simulink model "VisualLocalizationAgent"  (R2024b)
settings: Solver=FixedStepAuto  StartTime=0.0  StopTime=inf  FixedStep=0.005  RelTol=1e-3  EnableMultiTasking=on
undefined symbols (not defined in the file or in its folder): DiscIntNeverNeededParam, gray, Sim3dSensor
libraries: robotcorelib x7, dspstat3 x3, eeGeneralControl x2, sim3dcameralib x1, sim3dlib x1, uavsim3dlib x1, uavutilslib x1
settings Model: Creator=The MathWorks, Inc.  LastModifiedBy=Sasha
settings SolverCC: AlgebraicLoopSolver=TrustRegion  PositivePriorityOrder=on  AutoInsertRateTranBlk=on  MaxZcPerStep=1
settings OptimizationCC: DefaultParameterBehavior=Inlined  EnhancedBackFolding=on  PassReuseOutputArgsAs=Individual arguments  ZeroExternalMemoryAtStartup=off  ZeroInternalMemoryAtStartup=off  MaxStackSize=200000  OptimizeBlockOrder=speed  DifferentSizesBufferReuse=on  OptimizationCustomize=off  EfficientTunableParamExpr=on
settings DebuggingCC: ParameterTunabilityLossMsg=error  UnconnectedInputMsg=warning  UnconnectedOutputMsg=warning  UnconnectedLineMsg=warning  SymbolicDimsDataTypeCodeGenerationDiagnostic=none
settings HardwareCC: ProdBitPerPointer=32  ProdBitPerSizeT=32  ProdBitPerPtrDiffT=32  ProdLargestAtomicInteger=Long  ProdLargestAtomicFloat=Double  ProdWordSize=32  ProdLongLongMode=on  ProdHWDeviceType=ARM Compatible->ARM Cortex-A (32-bit)
settings ModelReferenceCC: EnableRefExpFcnMdlSchedulingChecks=on
settings RTWCC: Description=Embedded Coder  SystemTargetFile=ert.tlc  HardwareBoard=Raspberry Pi  TLCOptions="-aInlineSetEventsForThisBaseRateFcn=TLC_FALSE -aSuppressMultiTaskScheduler=TLC_FALSE  -aRateBasedStepFcn=0"  TemplateMakefile=ert_default_tmf  Toolchain=GNU GCC Embedded Linux  BuildConfiguration=Faster Runs  GPUComputeCapability=3.5  DLArmComputeVersion=19.05
settings CodeAppCC: ForceParamTrailComments=on  IgnoreCustomStorageClasses=off  OperatorAnnotations=on  SimulinkDataObjDesc=on  SFDataObjDesc=on  InsertBlockDesc=on
settings ERTTargetCC: CodeReplacementLibrary=ARM Cortex-A CMSIS  SupportVariableSizeSignals=on  ExtModeTransport=2  ExtModeStaticAlloc=on  ExtModeMexFile=ext_xcp  ExtModeIntrfLevel=Level2 - Open

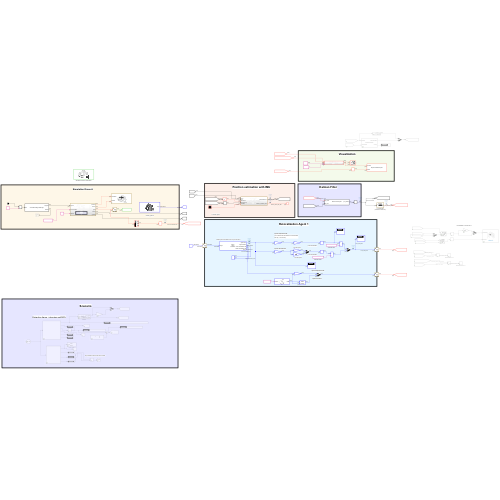
[thumbnail: Simulink's stored preview of the top-level diagram]
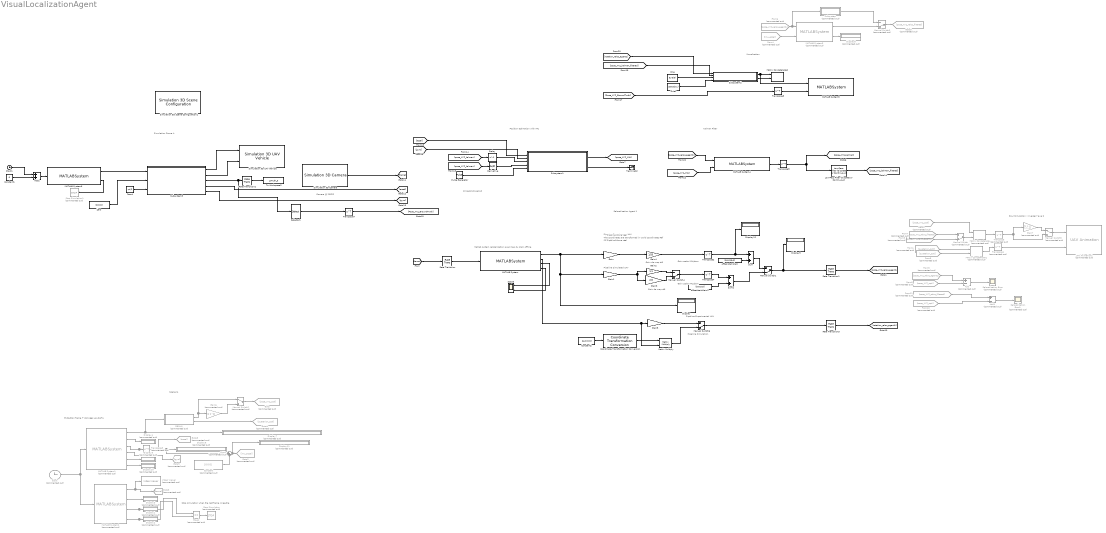
== system VisualLocalizationAgent ==
  note: Stop simulation when the last frame is reache
  note: Gain de map #6
  note: Pour Simulation : Inverser l'axe Z
  note: Pipeline Experimental UAV
  note: Matlab system relocalisation avec map du slam offline
  note: Gain scale IMU/slam
  note: Extraction frame + données uavDATA
  note: The coordinates are transformed in world coordinates
      |
      | Ref opti : (Y et Z inversé)
  note: Gain scale IMU/slam
  note: Pipeline drone réel
  note: Pipeline drone réel
  note: Pipeline Simulated UAV
  note: Gain de map #8
  note: 10 seconds period
  note: Relocalization Agent 1
  note: Scenario
  note: Position estimation with IMU
  note: Kalman Filter
  note: Visualization
  note: Camera @ 20FPS
  note: Simulation Drone A
  note: Pipeline Experimental UAV
  note: Pipeline Simulation
  Add : Sum  Commented=on  Inputs=+-
  Add1 : Sum  Commented=on  Inputs=+-
  Add2 : Sum
  Clock : Clock  Commented=on
  Clock1 : Clock
  Constant : Constant  Commented=on  Value=[0 0 0]
  Constant1 : Constant  Value=0
  Constant2 : Constant  Value=[pi/2;0;0]
  Coordinate Transformation Conversion : robotcorelib/Coordinate Transformation Conversion  InputRepresentation=Euler Angles  InputEulerSequence=ZYX  ShowTrVecInputPort=on  OutputRepresentation=Rotation Matrix  OutputEulerSequence=ZYX  ShowTrVecOutputPort=on  SimulateUsing=Code generation
  DEMUX : Subsystem  Commented=on
  Delay : Delay  DelayLength=1  InitialCondition=[0;0;0]
  Derivative : Derivative
  Display : Display
  Display{1..8,10..11} (10 alike) : Display  Commented=on
  Display12 : Display
  Display9 : Display
  Equal : RelationalOperator  Commented=on  Operator===  OutDataTypeStr=boolean  RndMeth=Simplest  InputSameDT=off
  From1 : From  Commented=on  GotoTag=quaterion_opti
  From10 : From  Commented=on  GotoTag=pose_XYZ_opti
  From11 : From  Commented=on  GotoTag=pose_XYZ_reloc_filtered
  From2 : From  Commented=on  GotoTag=pose_XYZ_opti
  From3 : From  Commented=on  GotoTag=pose_XYZ_reloc_agent1
  From4 : From  Commented=on  GotoTag=imu_accel
  From5 : From  Commented=on  GotoTag=quaterion_opti
  From6 : From  Commented=on  GotoTag=pose_XYZ_reloc_agent1
  From7 : From  Commented=on  GotoTag=pose_XYZ_reloc_filtered
  From8 : From  Commented=on  GotoTag=pose_XYZ_opti
  From9 : From  Commented=on  GotoTag=pose_XYZ_reloc_agent1
  Gain : Gain  Gain=[1 0 0; 0 -1 0 ; 0 0 -1]  Multiplication=Matrix(u*K)
  Gain1 : Gain  Gain=[0 -1 0; 1 0 0 ; 0 0 1]  Multiplication=Matrix(u*K)
  Gain2 : Gain  Gain=1.1
  Gain3 : Gain  Gain=2.6
  Gain4 : Gain  Gain=1/20
  Gain5 : Gain  Gain=[1 0 0; 0 -1 0 ; 0 0 -1]  Multiplication=Matrix(u*K)
  Gain6 : Gain  Commented=on  Gain=[1 1 -1]
  Gain7 : Gain  Commented=on  Gain=[1 1 -1; 1 1 -1]
  Goto : Goto  Commented=on  GotoTag=pose_XYZ_opti
  Goto2 : Goto  Commented=on  GotoTag=imu_accel
  Goto3 : Goto  Commented=on  GotoTag=frame
  Goto4 : Goto  Commented=on  GotoTag=quaterion_opti
  Goto5 : Goto  Commented=on  GotoTag=pose_XYZ_reloc_filtered
  Goto8 : Goto  Commented=on  GotoTag=accel
  Goto9 : Goto  Commented=on  GotoTag=gyro
  Low-Pass Filter (Discrete or Continuous) : eeGeneralControl/Low-Pass Filter (Discrete or Continuous)  K=1  T=0.05  B=inf  A=-inf  init_option=Inherited from block input  x0=0  Ts=-1
  MATLAB System : MATLABSystem  System=Modif_of_HelperVisualLocalizationSystem  FocalLength=[1109,1109]  PrincipalPoint=[640,360]  ImageSize=[720,1280]  ScaleFactor=1.2  NumLevels=8  NumPoints=2000  XLim=[-100 100]  YLim=[-100 100]  ZLim=[-100 100]  SampleTime=0.1  ScenariosDirectory=C:\Users\vince\Documents\SEN5\CollaborativeSLAM\Scenarios  ScenarioName=8
      mask Type: Modif_of_HelperVisualLocalizationSystem
      mask Display:
      | disp(['Helper' char(10) 'Visual' char(10) 'Localization']);
      | port_label('input',1,'Image');
      | port_label('output',1,'Agent Pose');
      | port_label('output',2,'Agent Rotation');
      | port_label('output',3,'Local relocalization fail');
      | port_label('output',4,'Global relocalization fail');
  MATLAB System1 : MATLABSystem  Commented=on  System=GTruthPlayerSystem  groundTruthFile=C:\Users\vince\Documents\SEN5\CollaborativeSLAM\Scenarios\7\uavData.mat  SimulateUsing=Interpreted execution
  MATLAB System2 : MATLABSystem  Commented=on  System=ImagePlayerSystem  imageFolder=C:\Users\vince\Documents\SEN5\CollaborativeSLAM\Scenarios\7\images  cameraSize=[720,1280, 1]  groundTruthFile=C:\Users\vince\Documents\SEN5\CollaborativeSLAM\Scenarios\7\uavData.mat  SimulateUsing=Interpreted execution
  MATLAB System3 : MATLABSystem  Commented=on  System=PositionAccelFilter  maxPositionJump=0.2  maxAcceleration=10.0  windowSize=5  alpha=0.1  SimulateUsing=Code generation
      mask Type: PositionAccelFilter
      mask Display:
      | disp('PositionAccelFilter');
      | port_label('input',1,'position');
      | port_label('input',2,'acceleration');
      | port_label('output',1,'filteredPosition');
      | port_label('output',2,'isJump');
  MATLAB System4 : MATLABSystem  System=KalmanFusionSystem  dt=0.1  noise_std=0.1  Q=0.001 * eye( 6 )  R=diag( [ 0.3, 0.3, 0.3, 0.1, 0.1, 0.1 ] )  SimulateUsing=Interpreted execution
  MATLAB System5 : MATLABSystem  System=HelperVisualizationSystem  XLim=[-10 50]  YLim=[-10 10]  ZLim=[-10 10]  SampleTime=-1  ScenariosDirectory=C:\Users\vince\Documents\SEN5\CollaborativeSLAM\Scenarios  ScenarioName=8  NumberOfPoses=1  SimulateUsing=Interpreted execution
      mask Type: HelperVisualizationSystem
      mask Display:
      | disp('HelperVisualizationSystem');
      | port_label('input',1,'TformID');
      | port_label('input',2,'Gtruth');
  MATLAB System6 : MATLABSystem  System=SmoothBasicWaypointManager  ScenariosDirectory=C:\Users\vince\Documents\SEN5\CollaborativeSLAM\Scenarios  ScenarioName=9a  StepTime=0.01  SimulateUsing=Interpreted execution
  Manual Switch : ManualSwitch  Commented=on  CurrentSetting=0
  Manual Switch1 : ManualSwitch  CurrentSetting=0
  Manual Switch2 : ManualSwitch  Commented=on
  Manual Switch3 : ManualSwitch  Commented=on  CurrentSetting=0
  Manual Switch4 : ManualSwitch  CurrentSetting=0
  Manual Switch5 : ManualSwitch  Commented=on
  Manual Switch6 : ManualSwitch  CurrentSetting=0
  Matrix Concatenate : Concatenate  Commented=on  Mode=Multidimensional array  ConcatenateDimension=2
  Matrix Concatenate1 : Concatenate  Commented=on  Mode=Multidimensional array  ConcatenateDimension=2
  Matrix Concatenate2 : Concatenate  Mode=Multidimensional array  ConcatenateDimension=2
  Matrix Multiply : Product  Multiplication=Matrix(*)
  One : Constant  Value=eye(3)  OutDataTypeStr=Inherit: Inherit via back propagation
  One1 : Constant  Value=zeros(3,1)  OutDataTypeStr=Inherit: Inherit via back propagation
  Pulse Generator : DiscretePulseGenerator  PulseType=Time based  Period=0.05  PulseWidth=50
  Rate Transition : RateTransition
  Rate Transition1 : RateTransition
  Rate Transition2 : RateTransition  OutPortSampleTime=0.01
  Rate Transition3 : RateTransition
  Relocalization Error : Scope  Commented=on
  Relocalization Error1 : Scope  Commented=on
  Scope : Scope  NumInputPorts=2
  Selector1 : Selector  InputPortWidth=7  IndexOptions=Index vector (dialog)  Indices=[1 2 3]  OutputSizes=1
  Simulation 3D Camera : sim3dcameralib/Simulation 3D Camera  Priority=1  sensorTag=Sim3dSensor�  sensorId=1  sensorName=Sim3dSensor�  vehTagList={'Scene Origin';'SimulinkVehicle1'}  vehTag=SimulinkVehicle1  mountLoc=Origin  offsetFlag=on  tmountOffset=[0.1, 0, 0.1]  extTmount=off  rmountOffset=[0, 0, 0]  extRmount=off  FocalLength=[1109, 1109]  OpticalCenter=[640, 360]  ImageSize=[720, 1280]  RadialDistortion=[0, 0]  TangentialDistortion=[0, 0]  SensorSkew=0  DepthOutportEnabled=off  SemanticOutportEnabled=off  TransformOutportEnabled=off  SampleTime=1/20  mountPoint=[0.1 0 0.1]  mountOrientation=[0 0 0]  aMode=3  ID=1
      settings: LibrarySourceBlock=drivingsim3d/Simulation 3D Camera
  Simulation 3D Scene Configuration1 : sim3dlib/Simulation 3D Scene Configuration  Priority=0  ProjectFormat=Default Scenes  SceneDesc=US city block  ProjectName=D:\Program Files\MATLAB\R2024b\toolbox\shared\sim3d_projects\automotive_project_windows\UE\WindowsNoEditor\VehicleSimulation.exe  ScenePath=/Game/Maps/USCityBlock  EnableOpenDRIVE=off  vehTagList={'Scene Origin';'SimulinkVehicle1'}  vehTag=SimulinkVehicle1  FreeCameraInitialTranslation=[0, 0, 0]  FreeCameraDefaultInitialTranslation=[-6, 0, 2]  FreeCameraInitialRotation=[0, 0, 0]  FreeCameraDefaultInitialRotation=[0, -15, 0]  OpVisEn=off  Ts=1/100  EnableWindow=on  EnableRemoteAccess=off  EnableWeather=off  SunAzimuth=90  SunAltitude=40.0  EnableGeospatialSun=off  Latitude=0  Longitude=0  Date=2023-01-01  Time=10:30:00  GeoTimeZone=-5.0  SunDaylightSaving=off  wind=1  clouds=10  EnableVolumetricClouds=off  CloudCoverage=0  CloudAltitude=6  fog=0  rain=0  RaindropsEffect=off  SnowDensity=0  EnableGeospatial=off  UseTrueOrigin=off  OriginHeight=200  OriginLatitude=40.744652  OriginLongitude=-73.988864  MapStyle=Aerial  AdditionalAssetIDs=[]  UseAdvancedSunSky=off  SolarTime=11  TimeZone=-5  Day=21  Month=9  Year=2022  UseDaylightSavingTime=on  DSTStartDay=10  DSTStartMonth=3  DSTEndDay=3  DSTEndMonth=11  DSTSwitchHour=2  sensorTag=MainCamera1  sensorId=1  sensorName=MainCamera1  mountLoc=Origin  offsetFlag=off  tmountOffset=[0, 0, 0]  rmountOffset=[0, 0, 0]  HorizontalResolution=1280  VerticalResolution=720  HorizontalFOV=60  mountPoint=[0 0 0]  mountOrientation=[0 0 0]  aMode=4  ID=1  GeoTrigger=Inactive
      settings: LibrarySourceBlock=uavsim3dlib/Simulation 3D Scene Configuration
  Simulation 3D UAV Vehicle : uavsim3dlib/Simulation 3D UAV Vehicle  Priority=-1  Mesh=Quadrotor  MeshPath=/MathWorksUAVContent/UAVs/HexaRotorUAV/HexaRotor.HexaRotor  Color=Black  ActorName=SimulinkVehicle1  UseGlobalFrame=off  InitialTranslation=[0 0 0]  InitialRotation=[0 0 0]  InitialTranslationGlobal=[0 0 0]  InitialGeoOrigin=[0 0 0]  InitialRotationGlobal=[0 0 0]  SampleTime=1/100  ActorType=SimulinkVehicle  ID=1  aMode=4  ActorTag=SimulinkVehicle1
  Stop Simulation : Stop  Commented=on
  Stop Simulation1 : Stop  Commented=on
  Subsystem : Subsystem  Commented=on
  Subsystem1 : Subsystem
  Subsystem2 : Subsystem
  Subsystem3 : Subsystem
  Sum : Sum
  Sum1 : Sum  Commented=on  Inputs=|++
  Sum2 : Sum
  Terminator : Terminator
  To Workspace2 : ToWorkspace  VariableName=gTruth_a  SaveFormat=Timeseries  SampleTime=-1
  Transpose : Math  Commented=on  Operator=transpose
  Transpose1 : Math  Commented=on  Operator=transpose
  Transpose{2,4..5,7..8} (5 alike) : Math  Operator=transpose
  Transpose3 : Math  Commented=on  Operator=transpose
  UAV Animation1 : uavutilslib/UAV Animation  Commented=on  NumUAV=2  DynamicUAVConfig=off  UAVType=Multirotor  UAVSize=0.1  UAVColor=[1 0 0]  UAVTrajectoryAlpha=1  InertialZDirection=Down  RotationFormat=Quaternion  DrawMarkers=off  SampleTime=-1
  Video Viewer : VideoViewer  Commented=on  colormapValue=gray(256)  FigPos=[184.333333333333 766.666666666667 706 510]
  Zero : Constant  Value=[0;0;0]  OutDataTypeStr=Inherit: Inherit via back propagation
  Zero4 : Constant  Value=-pi/2  OutDataTypeStr=Inherit: Inherit via back propagation
  offset start slam : Constant  Value=[0;0.33;0]
  offset start slam1 : Constant  Value=[0;0;3.5]
  wires:
  MATLAB System2/1 -> Goto3/1, Video Viewer/1
  MATLAB System/2 -> Matrix Multiply/2, Gain5/1  "Agent_Rotation"
  MATLAB System/1 -> Gain1/1, Display/1, Gain/1  "Agent_Translation_reloc"
  MATLAB System/3 -> Scope/1  "Local relocalization fail"
  MATLAB System/4 -> Scope/2  "Global relocalization fail"
  MATLAB System2/3 -> Equal/1, Display1/1
  Clock/1 -> MATLAB System2/1, MATLAB System1/1
  MATLAB System2/4 -> Equal/2, Display2/1
  MATLAB System2/2 -> Display3/1
  MATLAB System1/1 -> Display7/1, DEMUX/1(pose_refopti_gtruth)
  offset start slam/1 -> Sum/2
  Matrix Concatenate/1 -> Transpose/1
  Matrix Concatenate1/1 -> Transpose1/1
  Transpose/1 -> Gain7/1, Manual Switch5/2
  Transpose1/1 -> UAV Animation1/2
  From3/1 -> Manual Switch/2
  DEMUX/1(XYZ_gtruth) -> Manual Switch2/1, Gain6/1
  MATLAB System1/2 -> Display4/1
  MATLAB System1/5 -> Display5/1
  MATLAB System1/6 -> Display10/1
  MATLAB System1/3 -> Goto8/1, Transpose3/1
  Gain/1 -> Gain4/1
  Gain4/1 -> Transpose2/1
  Transpose2/1 -> Display12/1, Sum/1
  DEMUX/2(quaterion_gtruth) -> Goto4/1
  From1/1 -> Matrix Concatenate1/1
  From5/1 -> Matrix Concatenate1/2
  From4/1 -> MATLAB System3/2
  From6/1 -> Subsystem/1(In1), MATLAB System3/1
  From7/1 -> Manual Switch/1
  Manual Switch/1 -> Matrix Concatenate/2
  Transpose3/1 -> Sum1/1, Display6/1
  MATLAB System3/2 -> Display8/1
  Constant/1 -> Sum1/2
  Sum1/1 -> Display11/1, Goto2/1
  Sum/1 -> Manual Switch1/1
  MATLAB System3/1 -> Manual Switch3/2
  Subsystem/1(Out1) -> Manual Switch3/1
  Manual Switch1/1 -> Display9/1, Rate Transition1/1  "Pose_XYZ_Reloc"
  Gain1/1 -> Gain3/1, Gain2/1
  Transpose4/1 -> Sum2/1
  offset start slam1/1 -> Sum2/2
  Sum2/1 -> Manual Switch1/2
  From2/1 -> Matrix Concatenate/1
  Gain6/1 -> Manual Switch2/2
  Manual Switch2/1 -> Goto/1
  From8/1 -> Add/2  "Real_Pose_XYZ"
  Add/1 -> Relocalization Error/1  "Relocalization Error"
  From9/1 -> Add/1  "Estimated_Pose_XYZ"
  Add1/1 -> Relocalization Error1/1  "Filtered Relocalization Error"
  From10/1 -> Add1/2  "Real_Pose_XYZ"
  From11/1 -> Add1/1  "Estimated_Pose_XYZ_Filtered"
  Manual Switch3/1 -> Goto5/1
  Gain2/1 -> Manual Switch4/1
  Gain3/1 -> Manual Switch4/2
  Manual Switch4/1 -> Transpose4/1
  Equal/1 -> Stop Simulation/1
  Manual Switch5/1 -> UAV Animation1/1
  Gain7/1 -> Manual Switch5/1
  MATLAB System1/4 -> Goto9/1
  [gyro] -> Subsystem1/2(gyro)  "gyro"
  [accel] -> Subsystem1/1(accel)  "accel"
  Subsystem1/1(estimatedIMUPose) -> [pose_XYZ_IMU]  "pose_XYZ_IMU"
  Pulse Generator/1 -> Subsystem1/5(resetIMU)  "resetIMU"
  [pose_XYZ_kalman] -> Delay/1
  [pose_XYZ_reloc_agent1] -> MATLAB System4/1  "Estimated_Pose_XYZ"
  MATLAB System4/1 -> Transpose5/1
  [rotation_reloc_agent1] -> Subsystem2/1(In1)
  [pose_XYZ_kalman_filtered] -> Subsystem2/2(In2)
  Subsystem2/1(Out1) -> MATLAB System5/1, Matrix Concatenate2/1
  Subsystem2/2(Out2) -> Matrix Concatenate2/2
  Clock1/1 -> Add2/1
  Add2/1 -> MATLAB System6/1
  Subsystem3/4(accData) -> [accel]
  MATLAB System6/1 -> Subsystem3/1(waypoint)
  Zero/1 -> Subsystem3/2(translationOffset)
  Subsystem3/1(Translation) -> Simulation 3D UAV Vehicle/1
  Subsystem3/3(gTruth) -> Selector1/1, Rate Transition2/1
  Zero4/1 -> Subsystem3/3(initialYaw)
  Subsystem3/2(Rotation) -> Simulation 3D UAV Vehicle/2
  MATLAB System6/2 -> Stop Simulation1/1
  Constant1/1 -> Add2/2
  Subsystem3/5(gyroData) -> [gyro]
  Rate Transition2/1 -> To Workspace2/1
  Simulation 3D Camera/1 -> [frame]
  One1/1 -> Subsystem2/4(In4)
  One/1 -> Subsystem2/3(In3)
  [frame] -> Rate Transition/1
  [Pose_XYZ_GroundTruth] -> Transpose8/1
  Transpose5/1 -> Low-Pass Filter (Discrete or Continuous)/1, [pose_XYZ_kalman]  "Pose_XYZ_Kalman"
  Delay/1 -> Subsystem1/3(filteredPose)
  Selector1/1 -> Transpose7/1
  Transpose7/1 -> [Pose_XYZ_GroundTruth]  "Pose_XYZ_GroundTruth"
  Transpose8/1 -> MATLAB System5/2
  Subsystem1/2(Relative_Translation_XYZ) -> Terminator/1  "Relative_Pose_XYZ_IMU"
  [pose_XYZ_kalman] -> Derivative/1
  Derivative/1 -> Subsystem1/4(filteredVelocity)
  [pose_XYZ_IMU] -> MATLAB System4/2
  Rate Transition/1 -> MATLAB System/1
  Rate Transition1/1 -> [pose_XYZ_reloc_agent1]
  Rate Transition3/1 -> [rotation_reloc_agent1]
  Low-Pass Filter (Discrete or Continuous)/1 -> [pose_XYZ_kalman_filtered]  "Pose_XYZ_Kalman_filtered"
  Gain5/1 -> Manual Switch6/1
  Manual Switch6/1 -> Rate Transition3/1
  Constant2/1 -> Coordinate Transformation Conversion/1
  Coordinate Transformation Conversion/1 -> Matrix Multiply/1
  Matrix Multiply/1 -> Manual Switch6/2

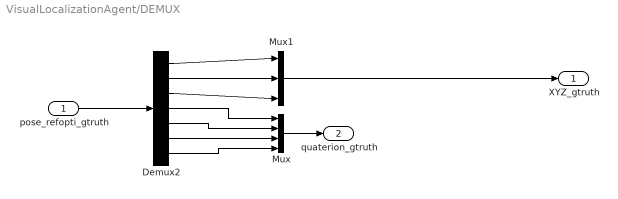
== system VisualLocalizationAgent/DEMUX ==
  pose_refopti_gtruth : Inport
  Demux2 : Demux  Outputs=7
  Mux : Mux
  Mux1 : Mux  Inputs=3
  XYZ_gtruth : Outport
  quaterion_gtruth : Outport  Port=2
  wires:
  Mux/1 -> quaterion_gtruth/1
  Demux2/2 -> Mux1/2
  Demux2/5 -> Mux/2
  Mux1/1 -> XYZ_gtruth/1
  Demux2/3 -> Mux1/3
  Demux2/4 -> Mux/1
  pose_refopti_gtruth/1 -> Demux2/1
  Demux2/7 -> Mux/4
  Demux2/6 -> Mux/3
  Demux2/1 -> Mux1/1

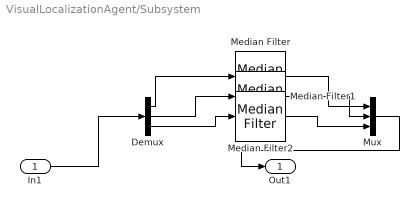
== system VisualLocalizationAgent/Subsystem ==
  In1 : Inport
  Demux : Demux  Outputs=3
  Median Filter : dspstat3/Median Filter  WindowLength=2  SimulateUsing=Interpreted execution
  Median Filter1 : dspstat3/Median Filter  WindowLength=2  SimulateUsing=Interpreted execution
  Median Filter2 : dspstat3/Median Filter  WindowLength=2  SimulateUsing=Interpreted execution
  Mux : Mux  Inputs=3
  Out1 : Outport  PortDimensions=[3 1]
  wires:
  Median Filter2/1 -> Mux/3
  In1/1 -> Demux/1
  Demux/3 -> Median Filter2/1
  Mux/1 -> Out1/1
  Demux/2 -> Median Filter1/1
  Demux/1 -> Median Filter/1
  Median Filter1/1 -> Mux/2
  Median Filter/1 -> Mux/1

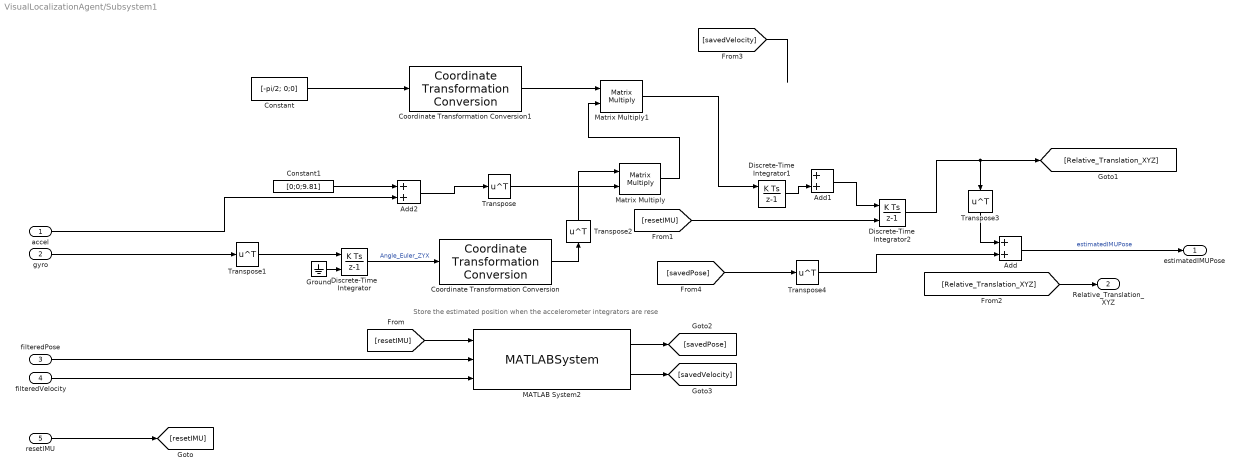
== system VisualLocalizationAgent/Subsystem1 ==
  note: Store the estimated position when the accelerometer integrators are rese
  accel : Inport
  gyro : Inport  Port=2
  filteredPose : Inport  Port=3
  filteredVelocity : Inport  Port=4  PortDimensions=[3,1]
  resetIMU : Inport  Port=5
  Add : Sum
  Add1 : Sum
  Add2 : Sum
  Constant : Constant  Value=[-pi/2; 0;0]
  Constant1 : Constant  Value=[0;0;9.81]
  Coordinate Transformation Conversion : robotcorelib/Coordinate Transformation Conversion  InputRepresentation=Euler Angles  InputEulerSequence=ZYX  ShowTrVecInputPort=on  OutputRepresentation=Rotation Matrix  OutputEulerSequence=ZYX  ShowTrVecOutputPort=on  SimulateUsing=Code generation
  Coordinate Transformation Conversion1 : robotcorelib/Coordinate Transformation Conversion  InputRepresentation=Euler Angles  InputEulerSequence=ZYX  ShowTrVecInputPort=on  OutputRepresentation=Rotation Matrix  OutputEulerSequence=ZYX  ShowTrVecOutputPort=on  SimulateUsing=Code generation
  Discrete-Time Integrator : DiscreteIntegrator  ExternalReset=rising  SampleTime=-1  ICPrevOutput=DiscIntNeverNeededParam  ICPrevScaledInput=DiscIntNeverNeededParam
  Discrete-Time Integrator1 : DiscreteIntegrator  ExternalReset=rising  SampleTime=-1  ICPrevOutput=DiscIntNeverNeededParam  ICPrevScaledInput=DiscIntNeverNeededParam
  Discrete-Time Integrator2 : DiscreteIntegrator  ExternalReset=rising  SampleTime=-1  ICPrevOutput=DiscIntNeverNeededParam  ICPrevScaledInput=DiscIntNeverNeededParam
  Ground : Ground
  MATLAB System2 : MATLABSystem  System=IMUPoseMemory  SimulateUsing=Interpreted execution
  Matrix Multiply : Product  Multiplication=Matrix(*)
  Matrix Multiply1 : Product  Multiplication=Matrix(*)
  Transpose{,1..4} (5 alike) : Math  Operator=transpose
  estimatedIMUPose : Outport
  Relative_Translation_XYZ : Outport  Port=2
  wires:
  filteredPose/1 -> MATLAB System2/2
  Transpose1/1 -> Discrete-Time Integrator/1
  [savedPose] -> Transpose4/1
  Constant1/1 -> Add2/1
  Discrete-Time Integrator1/1 -> Add1/2
  Ground/1 -> Discrete-Time Integrator/2
  [resetIMU] -> Discrete-Time Integrator2/2
  Coordinate Transformation Conversion/1 -> Transpose2/1
  Transpose/1 -> Matrix Multiply/2
  Add/1 -> estimatedIMUPose/1  "estimatedIMUPose"
  Discrete-Time Integrator/1 -> Coordinate Transformation Conversion/1  "Angle_Euler_ZYX"
  Add2/1 -> Transpose/1
  Transpose4/1 -> Add/2
  [resetIMU] -> MATLAB System2/1
  MATLAB System2/1 -> [savedPose]
  accel/1 -> Add2/2
  resetIMU/1 -> [resetIMU]
  gyro/1 -> Transpose1/1
  Constant/1 -> Coordinate Transformation Conversion1/1
  Coordinate Transformation Conversion1/1 -> Matrix Multiply1/1
  Discrete-Time Integrator2/1 -> Transpose3/1, [Relative_Translation_XYZ]
  Transpose2/1 -> Matrix Multiply/1
  [Relative_Translation_XYZ] -> Relative_Translation_XYZ/1
  filteredVelocity/1 -> MATLAB System2/3
  MATLAB System2/2 -> [savedVelocity]
  Add1/1 -> Discrete-Time Integrator2/1
  Transpose3/1 -> Add/1
  Matrix Multiply/1 -> Matrix Multiply1/2
  Matrix Multiply1/1 -> Discrete-Time Integrator1/1
  [savedVelocity] -> ?

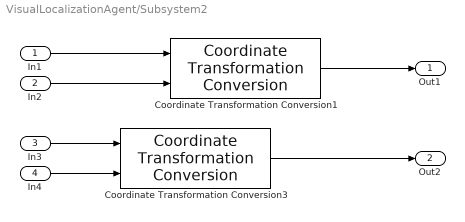
== system VisualLocalizationAgent/Subsystem2 ==
  In1 : Inport
  In2 : Inport  Port=2
  In3 : Inport  Port=3
  In4 : Inport  Port=4
  Coordinate Transformation Conversion1 : robotcorelib/Coordinate Transformation Conversion  InputRepresentation=Rotation Matrix  InputEulerSequence=ZYX  ShowTrVecInputPort=on  OutputRepresentation=Homogeneous Transformation  OutputEulerSequence=ZYX  ShowTrVecOutputPort=on  SimulateUsing=Code generation
      settings: LibrarySourceBlock=navlib/Utilities/Coordinate Transformation Conversion
  Coordinate Transformation Conversion3 : robotcorelib/Coordinate Transformation Conversion  InputRepresentation=Rotation Matrix  InputEulerSequence=ZYX  ShowTrVecInputPort=on  OutputRepresentation=Homogeneous Transformation  OutputEulerSequence=ZYX  ShowTrVecOutputPort=on  SimulateUsing=Code generation
      settings: LibrarySourceBlock=navlib/Utilities/Coordinate Transformation Conversion
  Out1 : Outport
  Out2 : Outport  Port=2
  wires:
  Coordinate Transformation Conversion3/1 -> Out2/1
  In3/1 -> Coordinate Transformation Conversion3/1
  Coordinate Transformation Conversion1/1 -> Out1/1
  In1/1 -> Coordinate Transformation Conversion1/1
  In4/1 -> Coordinate Transformation Conversion3/2
  In2/1 -> Coordinate Transformation Conversion1/2

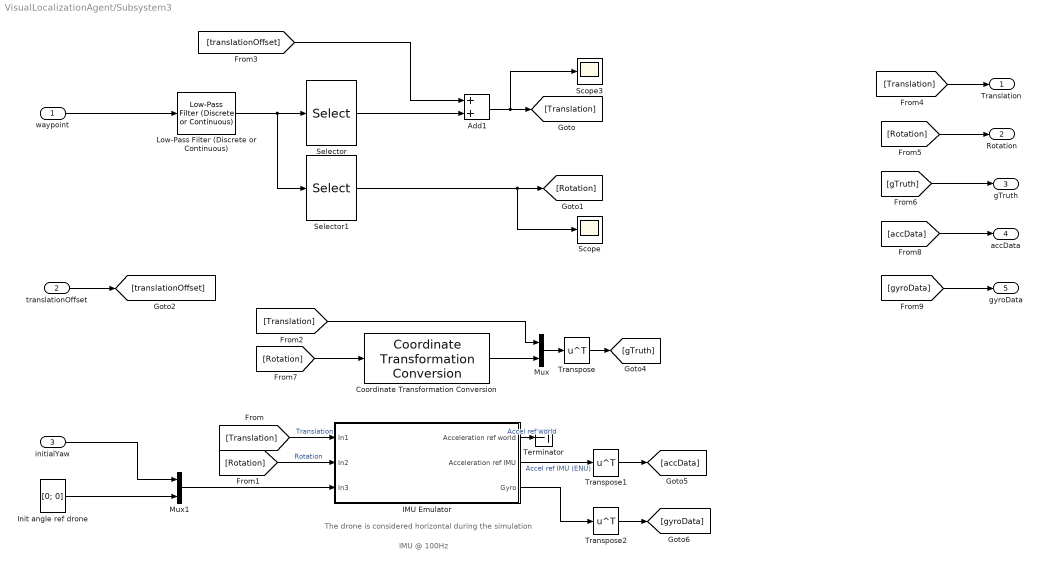
== system VisualLocalizationAgent/Subsystem3 ==
  note: IMU @ 100Hz
  note: The drone is considered horizontal during the simulation
  waypoint : Inport
  translationOffset : Inport  Port=2
  initialYaw : Inport  Port=3
  Add1 : Sum
  Coordinate Transformation Conversion : robotcorelib/Coordinate Transformation Conversion  InputRepresentation=Euler Angles  InputEulerSequence=ZYX  ShowTrVecInputPort=on  OutputRepresentation=Quaternion  OutputEulerSequence=ZYX  ShowTrVecOutputPort=on  SimulateUsing=Code generation
  IMU Emulator : Subsystem
  Init angle ref drone : Constant  Value=[0; 0]  VectorParams1D=off
  Low-Pass Filter (Discrete or Continuous) : eeGeneralControl/Low-Pass Filter (Discrete or Continuous)  K=1  T=0.5  B=inf  A=-inf  init_option=Inherited from block input  x0=0  Ts=-1
  Mux : Mux  Inputs=2
  Mux1 : Mux  Inputs=2
  Scope : Scope
  Scope3 : Scope
  Selector : Selector  InputPortWidth=6  IndexOptions=Index vector (dialog)  Indices=[1 2 3]  OutputSizes=1
  Selector1 : Selector  InputPortWidth=6  IndexOptions=Index vector (dialog)  Indices=[4 5 6]  OutputSizes=1
  Terminator : Terminator
  Transpose : Math  Operator=transpose
  Transpose1 : Math  Operator=transpose
  Transpose2 : Math  Operator=transpose
  Translation : Outport
  Rotation : Outport  Port=2
  gTruth : Outport  Port=3
  accData : Outport  Port=4
  gyroData : Outport  Port=5
  wires:
  waypoint/1 -> Low-Pass Filter (Discrete or Continuous)/1
  Add1/1 -> Scope3/1, [Translation]
  Transpose2/1 -> [gyroData]
  Selector/1 -> Add1/2
  Init angle ref drone/1 -> Mux1/2
  Selector1/1 -> [Rotation], Scope/1
  IMU Emulator/3(Gyro) -> Transpose2/1
  Coordinate Transformation Conversion/1 -> Mux/2
  IMU Emulator/1(Acceleration ref world) -> Terminator/1  "Accel ref world"
  [translationOffset] -> Add1/1
  Mux/1 -> Transpose/1
  [Rotation] -> Coordinate Transformation Conversion/1
  Transpose1/1 -> [accData]
  Transpose/1 -> [gTruth]
  [Translation] -> Mux/1
  Low-Pass Filter (Discrete or Continuous)/1 -> Selector1/1, Selector/1
  [Rotation] -> IMU Emulator/2(In2)  "Rotation"
  [Translation] -> IMU Emulator/1(In1)  "Translation"
  IMU Emulator/2(Acceleration ref IMU) -> Transpose1/1  "Accel ref IMU (ENU)"
  [Translation] -> Translation/1
  [Rotation] -> Rotation/1
  [gTruth] -> gTruth/1
  [accData] -> accData/1
  [gyroData] -> gyroData/1
  initialYaw/1 -> Mux1/1
  Mux1/1 -> IMU Emulator/3(In3)
  translationOffset/1 -> [translationOffset]

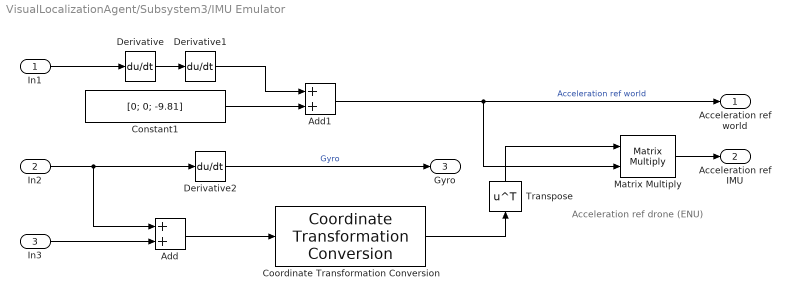
== system VisualLocalizationAgent/Subsystem3/IMU Emulator ==
  note: Acceleration ref drone (ENU)
  In1 : Inport
  In2 : Inport  Port=2
  In3 : Inport  Port=3
  Add : Sum
  Add1 : Sum
  Constant1 : Constant  Value=[0; 0; -9.81]
  Coordinate Transformation Conversion : robotcorelib/Coordinate Transformation Conversion  InputRepresentation=Euler Angles  InputEulerSequence=ZYX  ShowTrVecInputPort=on  OutputRepresentation=Rotation Matrix  OutputEulerSequence=ZYX  ShowTrVecOutputPort=on  SimulateUsing=Code generation
  Derivative : Derivative
  Derivative1 : Derivative
  Derivative2 : Derivative
  Matrix Multiply : Product  Multiplication=Matrix(*)
  Transpose : Math  Operator=transpose
  Acceleration ref world : Outport
  Acceleration ref IMU : Outport  Port=2
  Gyro : Outport  Port=3
  wires:
  Derivative/1 -> Derivative1/1
  Derivative2/1 -> Gyro/1  "Gyro"
  Constant1/1 -> Add1/2
  Add1/1 -> Matrix Multiply/2, Acceleration ref world/1  "Acceleration ref world"
  Derivative1/1 -> Add1/1
  In1/1 -> Derivative/1
  In2/1 -> Add/1, Derivative2/1
  In3/1 -> Add/2
  Add/1 -> Coordinate Transformation Conversion/1
  Matrix Multiply/1 -> Acceleration ref IMU/1
  Coordinate Transformation Conversion/1 -> Transpose/1
  Transpose/1 -> Matrix Multiply/1
